simulink model "Pneumatic Set Up Model Utilising 3_2 Solenoid Valves"  (R2021a)
settings: Solver=VariableStepAuto  StartTime=0.0  StopTime=1.346  RelTol=1e-3
undefined symbols (not defined in the file or in its folder): A_piston, A_rod, L_piston, sigbuilder_block, T_atm
libraries: fl_lib x25, nesl_utility x7, SimscapeFluids_lib x2
(part 2 of 2)

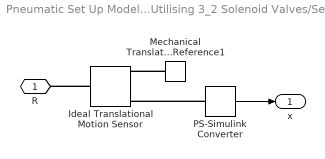
== system Pneumatic Set Up Model Utilising 3_2 Solenoid Valves/Sensor ==
  Ideal Translational Motion Sensor : fl_lib/Mechanical/Mechanical Sensors/Ideal Translational Motion Sensor  offset=0 m
  Mechanical Translational Reference1 : fl_lib/Mechanical/Translational Elements/Mechanical Translational Reference
  PS-Simulink Converter : nesl_utility/PS-Simulink Converter  PhysicalDomain=network_engine_domain  SubClassName=ps_output  LeftPortType=input  RightPortType=output  PseudoPeriodic=off  Frequencies=[]  Unit=m  AffineConversion=off
      settings: SourceProductBaseCode=PW,SS
  R : PMIOPort  Side=Left
  x : Outport  VectorParamsAs1DForOutWhenUnconnected=off
  wires:
  PS-Simulink Converter/1 -> x/1
  connections:
  Mechanical Translational Reference1/LConn1 -- Ideal Translational Motion Sensor/RConn1
  Ideal Translational Motion Sensor/LConn1 -- R/RConn1
  PS-Simulink Converter/LConn1 -- Ideal Translational Motion Sensor/RConn3

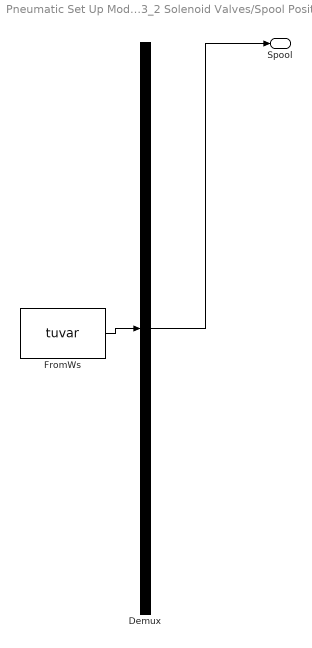
== system Pneumatic Set Up Model Utilising 3_2 Solenoid Valves/Spool Position ==
  Demux : Demux  Tag=STV Demux  Outputs=1
      settings: DisplayOption=none
  FromWs : FromWorkspace  Tag=STV FromWs  VariableName=tuvar
      SigBuilderData=|
      | common.afterFinalStr = 'Extrapolate'
      | common.sampleTime = 0
      | dataSet.timeRange = [0 1.346]
      | dataSet.name = 'Group 1'
      | sbobj.Groups.Name = 'Group 1'
      | sbobj.Groups.Signals.Name = 'Spool'
      | sbobj.Groups.Signals.XData = [0 0.025 0.1125 0.1375 0.4 0.425 0.666 0.691 0.791 0.816 1.0785 1.1035 1.346]
      | sbobj.Groups.Signals.YData = [0 5 5 -5 -5 -5 -5 5 5 -5 -5 -5 -5]
      | sbobj.Groups.TimeRange = [0 1.346]
  Spool : Outport  Tag=STV Outport  VectorParamsAs1DForOutWhenUnconnected=off
  wires:
  Demux/1 -> Spool/1
  FromWs/1 -> Demux/1

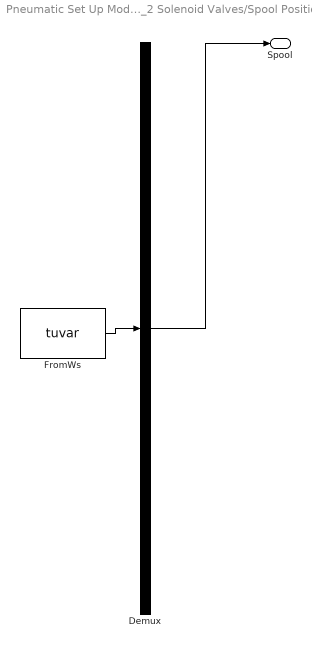
== system Pneumatic Set Up Model Utilising 3_2 Solenoid Valves/Spool Position1 ==
  Demux : Demux  Tag=STV Demux  Outputs=1
      settings: DisplayOption=none
  FromWs : FromWorkspace  Tag=STV FromWs  VariableName=tuvar
      SigBuilderData=|
      | common.afterFinalStr = 'Extrapolate'
      | common.sampleTime = 0
      | dataSet.timeRange = [0 1.346]
      | dataSet.name = 'Group 1'
      | sbobj.Groups.Name = 'Group 1'
      | sbobj.Groups.Signals.Name = 'Spool'
      | sbobj.Groups.Signals.XData = [0 0.025 0.1125 0.1375 0.35 0.375 0.666 0.691 0.791 0.816 1.0285 1.0535 1.33 1.346]
      | sbobj.Groups.Signals.YData = [-5 -5 -5 5 5.02 -5.02 -5 -5 -5 5 5 -5 -5 -5]
      | sbobj.Groups.TimeRange = [0 1.346]
  Spool : Outport  Tag=STV Outport  VectorParamsAs1DForOutWhenUnconnected=off
  wires:
  Demux/1 -> Spool/1
  FromWs/1 -> Demux/1
